simulink model "lab3miss"  (Simulink 7.9)
settings: Solver=ode45  StartTime=0.0  StopTime=150  RelTol=1e-3
settings Model: Creator=mkieler  LastModifiedBy=mkieler

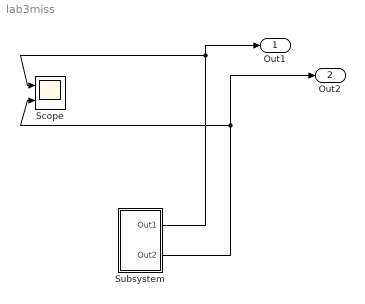
== system lab3miss ==
  Scope : Scope  NumInputPorts=2
      settings: TimeRange=4  YMin=-3.285211267605635~-5  YMax=0.7147887323943651~5
  Subsystem : Subsystem  mask{h1=4, h2=2, S1=1, S2=2, Swy1=0.2, Swy2=0.2, fi1=1, fi2=1, g=9.81, Qwe=2.8}
  Out1 : Outport
  Out2 : Outport  Port=2
  wires:
  Subsystem/1(Out1) -> Out1/1, Scope/1
  Subsystem/2(Out2) -> Out2/1, Scope/2

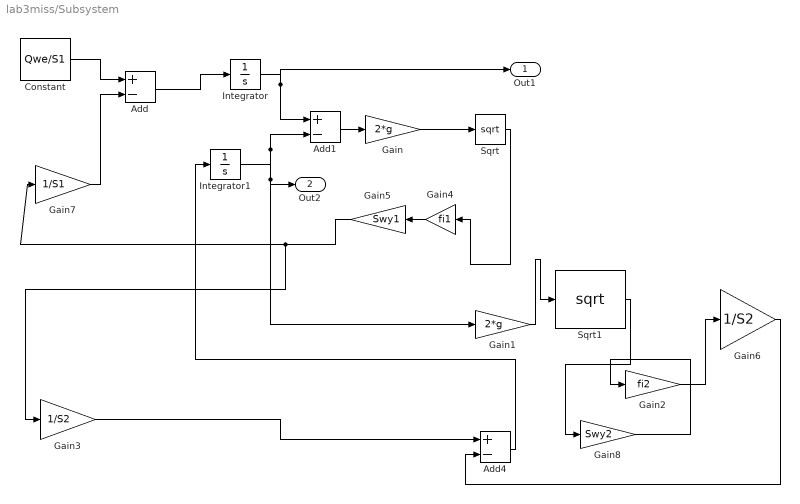
== system lab3miss/Subsystem ==
  Add : Sum  Inputs=+-
  Add1 : Sum  Inputs=+-
  Add4 : Sum  Inputs=+-
  Constant : Constant  Value=Qwe/S1
  Gain : Gain  Gain=2*g
  Gain1 : Gain  Gain=2*g
  Gain2 : Gain  Gain=fi2
  Gain3 : Gain  Gain=1/S2
  Gain4 : Gain  Gain=fi1
  Gain5 : Gain  Gain=Swy1
  Gain6 : Gain  Gain=1/S2
  Gain7 : Gain  Gain=1/S1
  Gain8 : Gain  Gain=Swy2
  Integrator : Integrator  InitialCondition=h1
  Integrator1 : Integrator  InitialCondition=h2
  Sqrt : Sqrt  SaturateOnIntegerOverflow=on
  Sqrt1 : Sqrt  SaturateOnIntegerOverflow=on
  Out1 : Outport
  Out2 : Outport  Port=2
  wires:
  Constant/1 -> Add/1
  Add/1 -> Integrator/1
  Integrator/1 -> Add1/1, Out1/1
  Integrator1/1 -> Add1/2, Gain1/1, Out2/1
  Add1/1 -> Gain/1
  Gain/1 -> Sqrt/1
  Sqrt/1 -> Gain4/1
  Gain4/1 -> Gain5/1
  Gain1/1 -> Sqrt1/1
  Gain5/1 -> Gain7/1, Gain3/1
  Gain2/1 -> Gain6/1
  Add4/1 -> Integrator1/1
  Gain3/1 -> Add4/1
  Gain6/1 -> Add4/2
  Sqrt1/1 -> Gain8/1
  Gain8/1 -> Gain2/1
  Gain7/1 -> Add/2
